simulink model "QuarterCar"  (R2024b)
settings: Solver=VariableStepAuto  StartTime=0.0  StopTime=10.0  RelTol=1e-3
libraries: fl_lib x7, nesl_utility x4
settings Model: Creator=Seb  LastModifiedBy=Seb

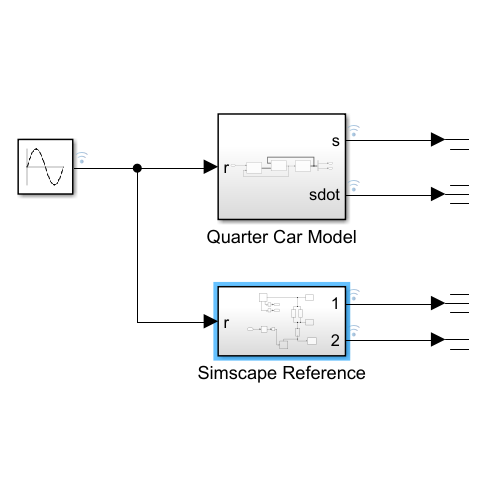
[thumbnail: Simulink's stored preview of the top-level diagram]
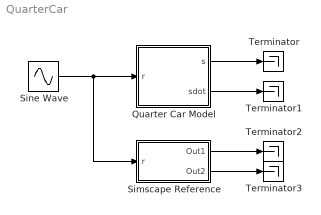
== system QuarterCar ==
  Quarter Car Model : Subsystem
  Simscape Reference : Subsystem
  Sine Wave : Sin  SampleTime=0
  Terminator{,1..3} (4 alike) : Terminator
  wires:
  Sine Wave/1 -> Simscape Reference/1(r), Quarter Car Model/1(r)
  Quarter Car Model/1(s) -> Terminator/1
  Quarter Car Model/2(sdot) -> Terminator1/1
  Simscape Reference/1(Out1) -> Terminator2/1
  Simscape Reference/2(Out2) -> Terminator3/1

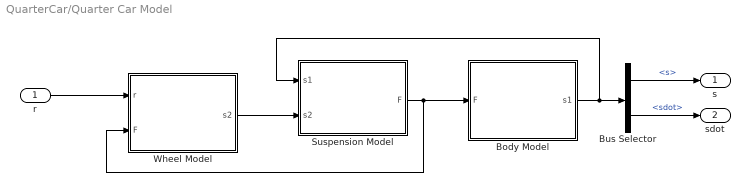
== system QuarterCar/Quarter Car Model ==
  r : Inport
  Body Model : Subsystem  mask{m1=250, g=9.81}
      mask prompts: m1 "Mass (m1)"; g "Gravity (g)"
      mask Display: fprintf("Body Model")
  Bus Selector : BusSelector  OutputSignals=s,sdot
  Suspension Model : Subsystem  mask{ks=20000, cs=1000}
      mask prompts: ks "Spring Stiffness (ks)"; cs "Damping Rate (cs)"
      mask Display: fprintf("Suspension\nModel")
  Wheel Model : Subsystem  mask{m2=20, g=9.81, kT=140000}
      mask prompts: m2 "Mass (m2)"; g "Gravity (g)"; kT "Wheel Stiffness (kT)"
      mask Display: fprintf("Wheel\nModel")
  s : Outport
  sdot : Outport  Port=2
  wires:
  Suspension Model/1(F) -> Wheel Model/2(F), Body Model/1(F)
  Wheel Model/1(s2) -> Suspension Model/2(s2)
  r/1 -> Wheel Model/1(r)
  Body Model/1(s1) -> Bus Selector/1, Suspension Model/1(s1)
  Bus Selector/1 -> s/1  "<s>"
  Bus Selector/2 -> sdot/1  "<sdot>"

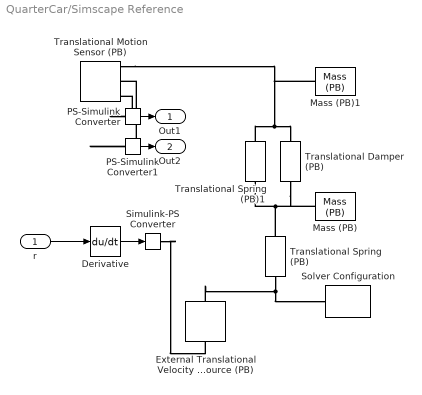
== system QuarterCar/Simscape Reference ==
  r : Inport
  Derivative : Derivative
  External Translational Velocity Source (PB) : fl_lib/Translational/Sources/External Translational Velocity Source (PB)  f_specify=off  f_priority=None  f=0 N  f_nominal_specify=off  f_nominal_value=1  f_nominal_unit=N
      settings: InternalSimscapePortConfiguration="{\"Bottom\":[],\"Left\":[],\"Right\":[{\"id\":\"R\",\"label\":\"R\",\"type\":\"foundation.translational.translational\"}],\"Top\":[{\"id\":\"S\",\"label\":\"S\",\"type\":\"input\"}]}"
  Mass (PB) : fl_lib/Translational/Elements/Mass (PB)  mass=25 kg  v_specify=off  v_priority=High  v=0 m/s  v_nominal_specify=off  v_nominal_value=1  v_nominal_unit=m/s  f_acc_specify=off  f_acc_priority=None  f_acc=0 N  f_acc_nominal_specify=off  f_acc_nominal_value=1  f_acc_nominal_unit=N  f_specify=off  f_priority=None  f=0 N  f_nominal_specify=off  f_nominal_value=1  f_nominal_unit=N
      settings: InternalSimscapePortConfiguration="{\"Bottom\":[],\"Left\":[{\"id\":\"R\",\"label\":\"R\",\"type\":\"foundation.translational.translational\"}],\"Right\":[],\"Top\":[]}"
  Mass (PB)1 : fl_lib/Translational/Elements/Mass (PB)  mass=250 kg  v_specify=off  v_priority=High  v=0 m/s  v_nominal_specify=off  v_nominal_value=1  v_nominal_unit=m/s  f_acc_specify=off  f_acc_priority=None  f_acc=0 N  f_acc_nominal_specify=off  f_acc_nominal_value=1  f_acc_nominal_unit=N  f_specify=off  f_priority=None  f=0 N  f_nominal_specify=off  f_nominal_value=1  f_nominal_unit=N
      settings: InternalSimscapePortConfiguration="{\"Bottom\":[],\"Left\":[{\"id\":\"R\",\"label\":\"R\",\"type\":\"foundation.translational.translational\"}],\"Right\":[],\"Top\":[]}"
  PS-Simulink Converter : nesl_utility/PS-Simulink Converter  PhysicalDomain=network_engine_domain  SubClassName=ps_output  LeftPortType=input  RightPortType=output  PseudoPeriodic=off  Frequencies=[]  VectorFormat=inherit  Unit=inherit  AffineConversion=off
  PS-Simulink Converter1 : nesl_utility/PS-Simulink Converter  PhysicalDomain=network_engine_domain  SubClassName=ps_output  LeftPortType=input  RightPortType=output  PseudoPeriodic=off  Frequencies=[]  VectorFormat=inherit  Unit=inherit  AffineConversion=off
  Simulink-PS Converter : nesl_utility/Simulink-PS Converter  PhysicalDomain=network_engine_domain  SubClassName=ps_input  LeftPortType=input  RightPortType=output  PseudoPeriodic=off  Frequencies=[]  NoiseDistribution=none  NoiseParameters=[]  Unit=1  AffineConversion=off  FilteringAndDerivatives=provide  SimscapeFilterOrder=1  InputFilterTimeConstant=0.001  UdotUserProvided=0
  Solver Configuration : nesl_utility/Solver Configuration  PhysicalDomain=network_engine_domain  SubClassName=solver  LeftPortType=input  RightPortType=generic  Tones=[]  Harmonics=[]  SimulateNoise=off  Profile=off  UseLocalSampling=off  EnableSwitchedLinearOptims=on  FrequencyDomain=off  UseCCode=off  RelTol=0.001  AbsTol=0.001  MinStep=1e-09  ToWorkspace=off  RevertToSquareIcSolve=off  NumHomotopyIterations=100  PhasorMode=off  PhasorModeNumHarmonics=1  ConsistencySolver=NEWTON_XTOL_AFTER_FTOL  IndexReductionMethod=DerivativeReplacement  DoDC=off  ResidualTolerance=1e-09  ConsistencyTolSource=GLOBAL  ConsistencyAbsTol=0.001  ConsistencyRelTol=0.001  ConsistencyTolFactor=0.001  UseLocalSolver=off  LocalSolverChoice=NE_BACKWARD_EULER_ADVANCER  ResolveIndetEquations=on  FunctionEvalNumThread=1  LocalSolverSampleTime=0.001  DoFixedCost=off  MaxNonlinIter=3  MaxModeIter=2  ComputeImpulses=off  ImpulseIterations=2  LinearAlgebra=auto  LinearAlgebraNumThread=0  EquationFormulation=NE_TIME_EF  DelaysMemoryBudget=1024  AutomaticFiltering=on  FilteringTimeConstant=0.001  PartitionStorageMethod=AS_NEEDED  PartitionMemoryBudget=1024  PartitionMethod=ROBUST  MultibodyUseLocalSolver=off  MultibodyLocalSolverChoice=ODE1  MultibodyLocalSolverSampleTime=0.001
  Translational Damper (PB) : fl_lib/Translational/Elements/Translational Damper (PB)  damping=1000 N*s/m  f_specify=off  f_priority=None  f=0 N  f_nominal_specify=off  f_nominal_value=1  f_nominal_unit=N  v_specify=off  v_priority=None  v=0 m/s  v_nominal_specify=off  v_nominal_value=1  v_nominal_unit=m/s  length_specify=off  length_priority=None  length=0 m  length_nominal_specify=off  length_nominal_value=1  length_nominal_unit=m
      settings: InternalSimscapePortConfiguration="{\"Bottom\":[],\"Left\":[{\"id\":\"B\",\"label\":\"B\",\"type\":\"foundation.translational.translational\"}],\"Right\":[{\"id\":\"F\",\"label\":\"F\",\"type\":\"foundation.translational.translational\"}],\"Top\":[]}"
  Translational Motion Sensor (PB) : fl_lib/Translational/Sensors/Translational Motion Sensor (PB)  reference=foundation.enum.MeasurementReference.absolute  acceleration_port=false  velocity_port=true  position_port=true
      settings: InternalSimscapePortConfiguration="{\"Bottom\":[{\"id\":\"V\",\"label\":\"V\",\"type\":\"output\"},{\"id\":\"P\",\"label\":\"P\",\"type\":\"output\"}],\"Left\":[],\"Right\":[{\"id\":\"F\",\"label\":\"F\",\"type\":\"foundation.translational.translational\"}],\"Top\":[]}"
  Translational Spring (PB) : fl_lib/Translational/Elements/Translational Spring (PB)  stiffness=14e4 N/m  f_specify=off  f_priority=None  f=0 N  f_nominal_specify=off  f_nominal_value=1  f_nominal_unit=N  deformation_specify=off  deformation_priority=None  deformation=0 m  deformation_nominal_specify=off  deformation_nominal_value=1  deformation_nominal_unit=m  length_specify=off  length_priority=None  length=0.1 m  length_nominal_specify=off  length_nominal_value=1  length_nominal_unit=m  rest_length_specify=off  rest_length_priority=None  rest_length=0.1 m  rest_length_nominal_specify=off  rest_length_nominal_value=1  rest_length_nominal_unit=m
      settings: InternalSimscapePortConfiguration="{\"Bottom\":[],\"Left\":[{\"id\":\"B\",\"label\":\"B\",\"type\":\"foundation.translational.translational\"}],\"Right\":[{\"id\":\"F\",\"label\":\"F\",\"type\":\"foundation.translational.translational\"}],\"Top\":[]}"
  Translational Spring (PB)1 : fl_lib/Translational/Elements/Translational Spring (PB)  stiffness=2e4 N/m  f_specify=off  f_priority=None  f=0 N  f_nominal_specify=off  f_nominal_value=1  f_nominal_unit=N  deformation_specify=off  deformation_priority=None  deformation=0 m  deformation_nominal_specify=off  deformation_nominal_value=1  deformation_nominal_unit=m  length_specify=off  length_priority=None  length=0.1 m  length_nominal_specify=off  length_nominal_value=1  length_nominal_unit=m  rest_length_specify=off  rest_length_priority=None  rest_length=0.1 m  rest_length_nominal_specify=off  rest_length_nominal_value=1  rest_length_nominal_unit=m
      settings: InternalSimscapePortConfiguration="{\"Bottom\":[],\"Left\":[{\"id\":\"B\",\"label\":\"B\",\"type\":\"foundation.translational.translational\"}],\"Right\":[{\"id\":\"F\",\"label\":\"F\",\"type\":\"foundation.translational.translational\"}],\"Top\":[]}"
  Out1 : Outport
  Out2 : Outport  Port=2
  wires:
  r/1 -> Derivative/1
  PS-Simulink Converter/1 -> Out1/1
  PS-Simulink Converter1/1 -> Out2/1
  Derivative/1 -> Simulink-PS Converter/1
  connections:
  Translational Spring (PB)/RConn1 -- External Translational Velocity Source (PB)/RConn1 -- Solver Configuration/RConn1
  Translational Spring (PB)/LConn1 -- Mass (PB)/LConn1 -- Translational Damper (PB)/RConn1 -- Translational Spring (PB)1/RConn1
  Translational Spring (PB)1/LConn1 -- Mass (PB)1/LConn1 -- Translational Motion Sensor (PB)/RConn1 -- Translational Damper (PB)/LConn1
  PS-Simulink Converter/LConn1 -- Translational Motion Sensor (PB)/RConn3
  PS-Simulink Converter1/LConn1 -- Translational Motion Sensor (PB)/RConn2
  Simulink-PS Converter/RConn1 -- External Translational Velocity Source (PB)/LConn1

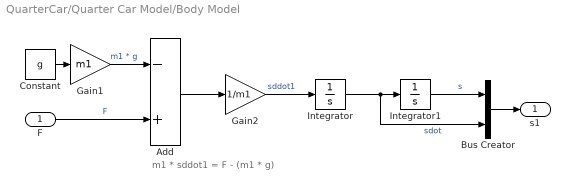
== system QuarterCar/Quarter Car Model/Body Model ==
  note: m1 * sddot1 = F - (m1 * g)
  F : Inport
  Add : Sum  Inputs=-+
  Bus Creator : BusCreator  Inputs=2
  Constant : Constant  Value=g
  Gain1 : Gain  Gain=m1
  Gain2 : Gain  Gain=1/m1
  Integrator : Integrator
  Integrator1 : Integrator
  s1 : Outport
  wires:
  F/1 -> Add/2  "F"
  Integrator1/1 -> Bus Creator/1  "s"
  Integrator/1 -> Bus Creator/2, Integrator1/1  "sdot"
  Add/1 -> Gain2/1
  Constant/1 -> Gain1/1
  Gain1/1 -> Add/1  "m1 * g"
  Gain2/1 -> Integrator/1  "sddot1"
  Bus Creator/1 -> s1/1

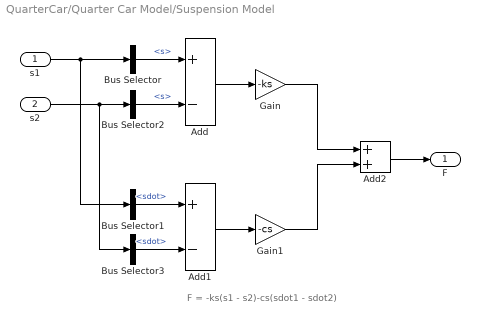
== system QuarterCar/Quarter Car Model/Suspension Model ==
  note: F = -ks(s1 - s2)-cs(sdot1 - sdot2)
  s1 : Inport
  s2 : Inport  Port=2
  Add : Sum  Inputs=+-
  Add1 : Sum  Inputs=+-
  Add2 : Sum
  Bus Selector : BusSelector  OutputSignals=s
  Bus Selector1 : BusSelector  OutputSignals=sdot
  Bus Selector2 : BusSelector  OutputSignals=s
  Bus Selector3 : BusSelector  OutputSignals=sdot
  Gain : Gain  Gain=-ks
  Gain1 : Gain  Gain=-cs
  F : Outport
  wires:
  s1/1 -> Bus Selector1/1, Bus Selector/1
  s2/1 -> Bus Selector3/1, Bus Selector2/1
  Add/1 -> Gain/1
  Bus Selector/1 -> Add/1  "<s>"
  Bus Selector1/1 -> Add1/1  "<sdot>"
  Add1/1 -> Gain1/1
  Gain/1 -> Add2/1
  Gain1/1 -> Add2/2
  Add2/1 -> F/1
  Bus Selector2/1 -> Add/2  "<s>"
  Bus Selector3/1 -> Add1/2  "<sdot>"

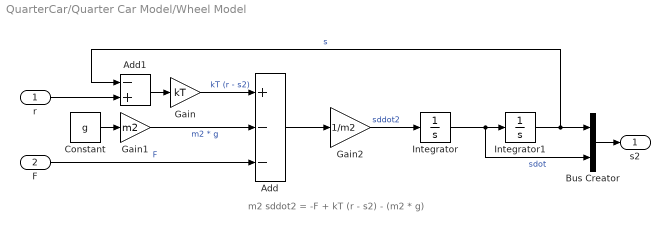
== system QuarterCar/Quarter Car Model/Wheel Model ==
  note: m2 sddot2 = -F + kT (r - s2) - (m2 * g)
  r : Inport
  F : Inport  Port=2
  Add : Sum  Inputs=+--
  Add1 : Sum  Inputs=-+
  Bus Creator : BusCreator  Inputs=2
  Constant : Constant  Value=g
  Gain : Gain  Gain=kT
  Gain1 : Gain  Gain=m2
  Gain2 : Gain  Gain=1/m2
  Integrator : Integrator
  Integrator1 : Integrator
  s2 : Outport
  wires:
  r/1 -> Add1/2
  Bus Creator/1 -> s2/1
  Gain2/1 -> Integrator/1  "sddot2"
  Constant/1 -> Gain1/1
  Integrator/1 -> Bus Creator/2, Integrator1/1  "sdot"
  Add/1 -> Gain2/1
  Integrator1/1 -> Add1/1, Bus Creator/1  "s"
  Gain1/1 -> Add/2  "m2 * g"
  F/1 -> Add/3  "F"
  Gain/1 -> Add/1  "kT (r - s2)"
  Add1/1 -> Gain/1
